simulink model "slip_regulation_stage2"  (R2018a)
settings: Solver=ode4  StartTime=0.0  StopTime=100  FixedStep=0.001  RelTol=1e-3
values from neighbouring files (symbols this model uses):
  B0 = 2.5    [init_params.m]
  Is = 0.2    [init_params.m]
  m = 100    [init_params.m]
  MFC1 = [9.5 1.9 1.14  0.75]    [init_params.m]
  MFC2 = [2.5 1.8 1 0.2]    [init_params.m]
  MFC3 = [1.5 1.8 0.4 0.2]    [init_params.m]
  N = 500    [init_params.m]
  r = 0.2    [init_params.m]
  v0 = 1    [init_params.m]
libraries: simulink x1
settings Model: Creator=obrusvit  LastModifiedBy=obrusvit

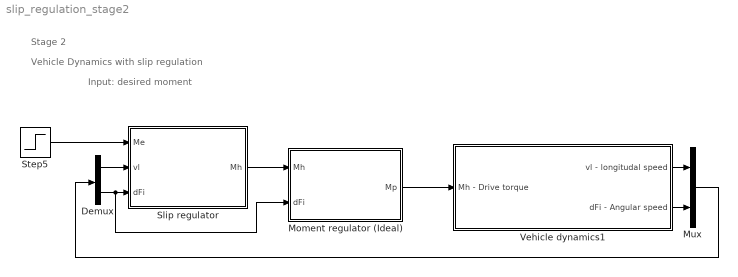
== system slip_regulation_stage2 ==
  note: Stage 2
  note: Input: desired moment
  note: Vehicle Dynamics with slip regulation
  Demux : Demux  Outputs=2
  Moment regulator (Ideal) : Subsystem
  Mux : Mux  Inputs=2
  Slip regulator : Subsystem
  Step5 : Step  Time=0  After=125  SampleTime=0
  Vehicle dynamics1 : Subsystem
  wires:
  Moment regulator (Ideal)/1("Mp ") -> Vehicle dynamics1/1(Mh - Drive torque)
  Slip regulator/1("Mh ") -> Moment regulator (Ideal)/1(Mh)
  Vehicle dynamics1/2(dFi - Angular speed) -> Mux/2
  Step5/1 -> Slip regulator/1(Me)
  Vehicle dynamics1/1(vl - longitudal speed) -> Mux/1
  Mux/1 -> Demux/1
  Demux/1 -> Slip regulator/2(vl)
  Demux/2 -> Moment regulator (Ideal)/2(dFi), Slip regulator/3(dFi)

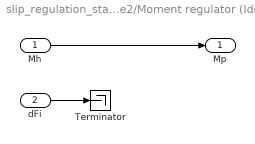
== system slip_regulation_stage2/Moment regulator (Ideal) ==
  Mh : Inport
  dFi : Inport  Port=2
  Terminator : Terminator
  "Mp " : Outport
  wires:
  Mh/1 -> "Mp "/1
  dFi/1 -> Terminator/1

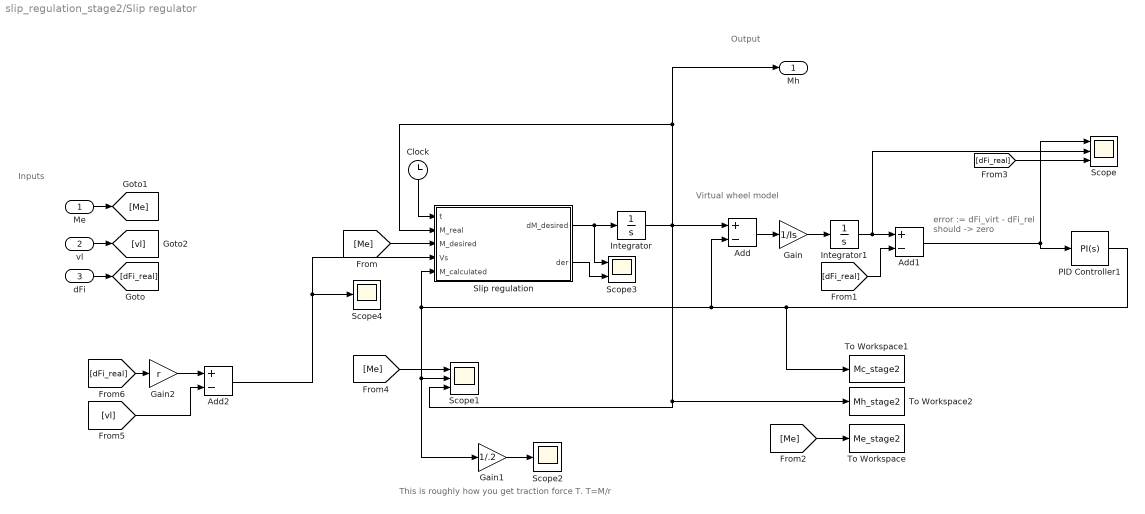
== system slip_regulation_stage2/Slip regulator ==
  note: This is roughly how you get traction force T. T=M/r
  note: error := dFi_virt - dFi_rel
      | should -> zero
  note: Virtual wheel model
  note: Output
  note: Inputs
  Me : Inport
  vl : Inport  Port=2
  dFi : Inport  Port=3
  Add : Sum  Inputs=+-
  Add1 : Sum  Inputs=+-
  Add2 : Sum  Inputs=+-
  Clock : Clock
  Gain : Gain  Gain=1/Is
  Gain1 : Gain  Gain=1/.2
  Gain2 : Gain  Gain=r
  Integrator : Integrator  LimitOutput=on  LowerSaturationLimit=0
  Integrator1 : Integrator
  PID Controller1 : simulink/Continuous/PID Controller  Controller=PI  TimeDomain=Continuous-time  SampleTime=-1  IntegratorMethod=Forward Euler  FilterMethod=Forward Euler  Form=Parallel  UseFilter=on  ControllerParametersSource=internal  P=15  I=20  D=0  N=100  InitialConditionSource=internal  InitialConditionForIntegrator=0  InitialConditionForFilter=0  ExternalReset=none  LimitOutput=on  UpperSaturationLimit=inf  LowerSaturationLimit=0  LinearizeAsGain=on  AntiWindupMode=none  Kb=1  TrackingMode=off  Kt=1  PParamMin=[]  PParamMax=[]  IParamMin=[]  IParamMax=[]  DParamMin=[]  DParamMax=[]  NParamMin=[]  NParamMax=[]  KbParamMin=[]  KbParamMax=[]  KtParamMin=[]  KtParamMax=[]  POutMin=[]  POutMax=[]  IOutMin=[]  IOutMax=[]  DOutMin=[]  DOutMax=[]  NOutMin=[]  NOutMax=[]  KbOutMin=[]  KbOutMax=[]  KtOutMin=[]  KtOutMax=[]  IntegratorOutMin=[]  IntegratorOutMax=[]  FilterOutMin=[]  FilterOutMax=[]  SumOutMin=[]  SumOutMax=[]  SumI1OutMin=[]  SumI1OutMax=[]  SumI2OutMin=[]  SumI2OutMax=[]  SumI3OutMin=[]  SumI3OutMax=[]  SumDOutMin=[]  SumDOutMax=[]  SaturationOutMin=[]  SaturationOutMax=[]  IntegratorContinuousStateAttributes=''  IntegratorStateMustResolveToSignalObject=off  IntegratorRTWStateStorageClass=Auto  FilterContinuousStateAttributes=''  FilterStateMustResolveToSignalObject=off  FilterRTWStateStorageClass=Auto  DifferentiatorICPrevScaledInput=0  DifferentiatorOutMin=[]  DifferentiatorOutMax=[]  FilterDiffOutCoefMin=[]  FilterDiffOutCoefMax=[]  SumDenOutMin=[]  SumDenOutMax=[]  SumNumOutMin=[]  SumNumOutMax=[]  ReciprocalOutMin=[]  ReciprocalOutMax=[]  DivideOutMin=[]  DivideOutMax=[]  TunerSelectOption=Transfer Function Based (PID Tuner App)
  Scope : Scope  NumInputPorts=3
  Scope1 : Scope  NumInputPorts=3
  Scope2 : Scope
  Scope3 : Scope  NumInputPorts=2
  Scope4 : Scope
  Slip regulation : MATLAB Function  TreatAsAtomicUnit=on
  To Workspace : ToWorkspace  VariableName=Me_stage2  SaveFormat=Timeseries  SampleTime=-1
  To Workspace1 : ToWorkspace  VariableName=Mc_stage2  SaveFormat=Timeseries  SampleTime=-1
  To Workspace2 : ToWorkspace  VariableName=Mh_stage2  SaveFormat=Timeseries  SampleTime=-1
  "Mh " : Outport
  wires:
  dFi/1 -> [dFi_real]
  Me/1 -> [Me]
  [Me] -> Slip regulation/3(M_desired)
  Slip regulation/1(dM_desired) -> Integrator/1, Scope3/1
  Add/1 -> Gain/1
  Gain/1 -> Integrator1/1
  [dFi_real] -> Add1/2
  Add1/1 -> PID Controller1/1, Scope/1
  Integrator1/1 -> Scope/2, Add1/1
  [dFi_real] -> Scope/3
  PID Controller1/1 -> To Workspace1/1, Scope1/2, Gain1/1, Slip regulation/5(M_calculated), Add/2
  [Me] -> Scope1/1
  Gain1/1 -> Scope2/1
  vl/1 -> [vl]
  Gain2/1 -> Add2/1
  [vl] -> Add2/2
  Add2/1 -> Scope4/1, Slip regulation/4(Vs)
  Clock/1 -> Slip regulation/1(t)
  Slip regulation/2(der) -> Scope3/2
  Integrator/1 -> Slip regulation/2(M_real), "Mh "/1, To Workspace2/1, Scope1/3, Add/1
  [dFi_real] -> Gain2/1
  [Me] -> To Workspace/1

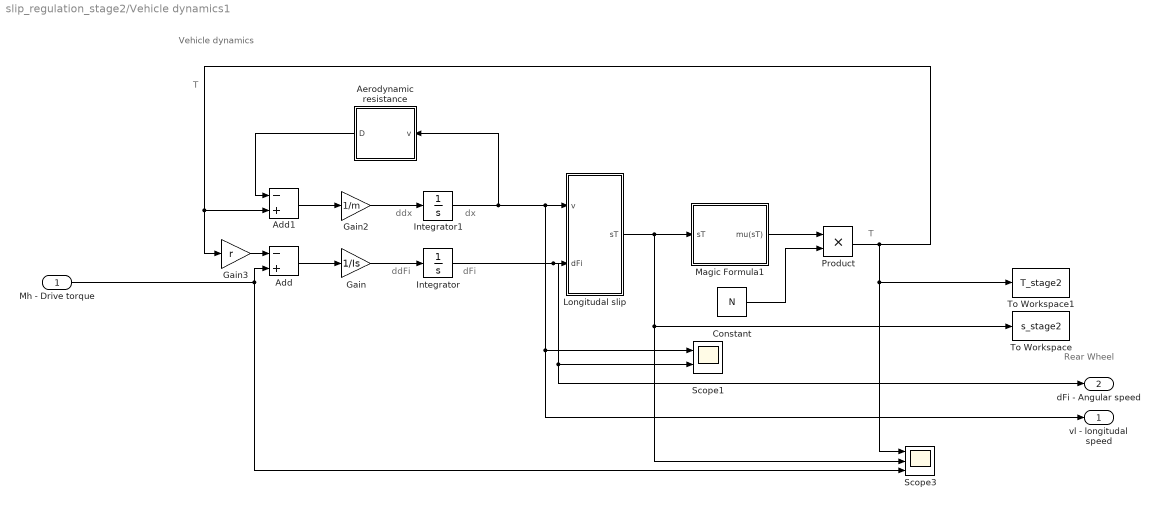
== system slip_regulation_stage2/Vehicle dynamics1 ==
  note: Vehicle dynamics
  note: Rear Wheel
  note: T
  note: ddx
  note: dx
  note: ddFi
  note: T
  note: dFi
  Mh - Drive torque : Inport
  Add : Sum  Inputs=-+
  Add1 : Sum  Inputs=-+
  "Aerodynamic resistance " : Subsystem
  Constant : Constant  Value=N
  Gain : Gain  Gain=1/Is
  Gain2 : Gain  Gain=1/m
  Gain3 : Gain  Gain=r
  Integrator : Integrator  InitialCondition=v0/r
  Integrator1 : Integrator  InitialCondition=v0
  Longitudal slip : Subsystem
  Magic Formula1 : Subsystem
  Product : Product
  Scope1 : Scope  NumInputPorts=2
  Scope3 : Scope  NumInputPorts=3
  To Workspace : ToWorkspace  VariableName=s_stage2  SaveFormat=Timeseries  SampleTime=-1
  To Workspace1 : ToWorkspace  VariableName=T_stage2  SaveFormat=Timeseries  SampleTime=-1
  vl - longitudal speed : Outport
  dFi - Angular speed : Outport  Port=2
  wires:
  Add1/1 -> Gain2/1
  Product/1 -> Gain3/1, Add1/2, To Workspace1/1, Scope3/1
  "Aerodynamic resistance "/1("D ") -> Add1/1
  Gain3/1 -> Add/1
  Magic Formula1/1(mu(sT)) -> Product/1
  Gain/1 -> Integrator/1
  Add/1 -> Gain/1
  Mh - Drive torque/1 -> Scope3/3, Add/2
  Constant/1 -> Product/2
  Gain2/1 -> Integrator1/1
  Integrator1/1 -> "Aerodynamic resistance "/1(v), Longitudal slip/1(v), vl - longitudal speed/1, Scope1/1
  Integrator/1 -> Scope1/2, dFi - Angular speed/1, Longitudal slip/2(dFi)
  Longitudal slip/1(sT) -> Scope3/2, To Workspace/1, Magic Formula1/1(sT)

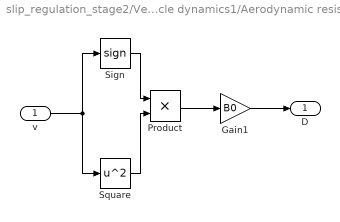
== system slip_regulation_stage2/Vehicle dynamics1/Aerodynamic resistance  ==
  v : Inport
  Gain1 : Gain  Gain=B0
  Product : Product
  Sign : Signum
  Square : Math  Operator=square  SaturateOnIntegerOverflow=on
  "D " : Outport
  wires:
  v/1 -> Sign/1, Square/1
  Square/1 -> Product/2
  Sign/1 -> Product/1
  Gain1/1 -> "D "/1
  Product/1 -> Gain1/1

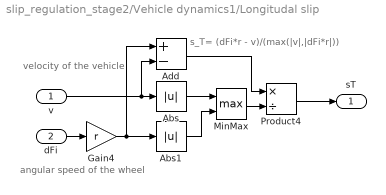
== system slip_regulation_stage2/Vehicle dynamics1/Longitudal slip ==
  note: s_T= (dFi*r - v)/(max(|v|,|dFi*r|))
  note: angular speed
      | of the wheel
  note: velocity
      | of the vehicle
  v : Inport
  dFi : Inport  Port=2
  Abs : Abs
  Abs1 : Abs
  Add : Sum  Inputs=+-
  Gain4 : Gain  Gain=r
  MinMax : MinMax  Function=max  Inputs=2
  Product4 : Product  Inputs=*/  RndMeth=Zero
  sT : Outport
  wires:
  Product4/1 -> sT/1
  Add/1 -> Product4/1
  Abs1/1 -> MinMax/2
  Abs/1 -> MinMax/1
  MinMax/1 -> Product4/2
  Gain4/1 -> Add/1, Abs1/1
  dFi/1 -> Gain4/1
  v/1 -> Add/2, Abs/1

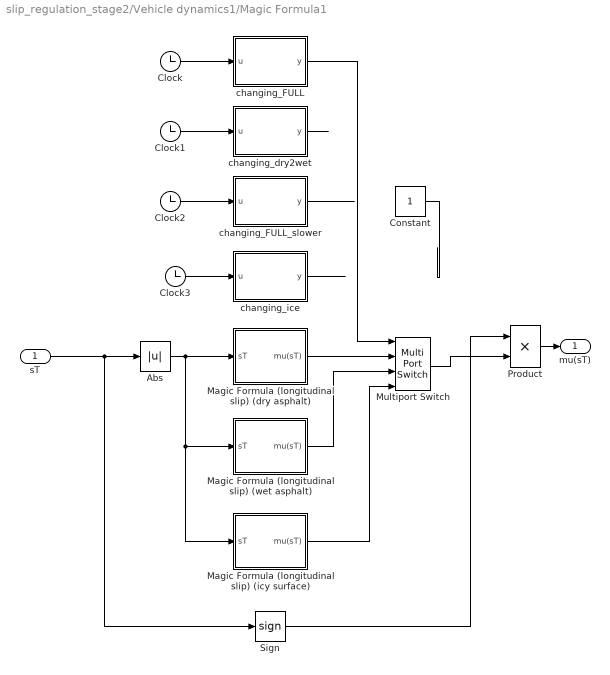
== system slip_regulation_stage2/Vehicle dynamics1/Magic Formula1 ==
  sT : Inport
  Abs : Abs
  Clock{,1..3} (4 alike) : Clock
  Constant : Constant
  Magic Formula (longitudinal slip) (dry asphalt) : Subsystem
  Magic Formula (longitudinal slip) (icy surface) : Subsystem
  Magic Formula (longitudinal slip) (wet asphalt) : Subsystem
  Multiport Switch : MultiPortSwitch
  Product : Product
  Sign : Signum
  changing_FULL : MATLAB Function  TreatAsAtomicUnit=on
  changing_FULL_slower : MATLAB Function  TreatAsAtomicUnit=on
  changing_dry2wet : MATLAB Function  TreatAsAtomicUnit=on
  changing_ice : MATLAB Function  TreatAsAtomicUnit=on
  mu(sT) : Outport
  wires:
  Abs/1 -> Magic Formula (longitudinal slip) (icy surface)/1(sT), Magic Formula (longitudinal slip) (wet asphalt)/1(sT), Magic Formula (longitudinal slip) (dry asphalt)/1(sT)
  Magic Formula (longitudinal slip) (dry asphalt)/1(mu(sT)) -> Multiport Switch/2
  Product/1 -> mu(sT)/1
  Sign/1 -> Product/1
  sT/1 -> Sign/1, Abs/1
  Magic Formula (longitudinal slip) (wet asphalt)/1(mu(sT)) -> Multiport Switch/3
  Multiport Switch/1 -> Product/2
  Magic Formula (longitudinal slip) (icy surface)/1(mu(sT)) -> Multiport Switch/4
  Clock/1 -> changing_FULL/1(u)
  changing_FULL/1(y) -> Multiport Switch/1
  Constant/1 -> ?
  Clock1/1 -> changing_dry2wet/1(u)
  changing_dry2wet/1(y) -> ?
  Clock2/1 -> changing_FULL_slower/1(u)
  changing_FULL_slower/1(y) -> ?
  changing_ice/1(y) -> ?
  Clock3/1 -> changing_ice/1(u)

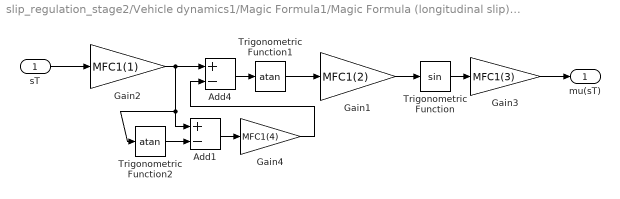
== system slip_regulation_stage2/Vehicle dynamics1/Magic Formula1/Magic Formula (longitudinal slip) (dry asphalt) ==
  sT : Inport
  Add1 : Sum  Inputs=+-
  Add4 : Sum  Inputs=+-
  Gain1 : Gain  Gain=MFC1(2)
  Gain2 : Gain  Gain=MFC1(1)
  Gain3 : Gain  Gain=MFC1(3)
  Gain4 : Gain  Gain=MFC1(4)
  Trigonometric Function : Trigonometry
  Trigonometric Function1 : Trigonometry  Operator=atan
  Trigonometric Function2 : Trigonometry  Operator=atan
  mu(sT) : Outport
  wires:
  Gain3/1 -> mu(sT)/1
  sT/1 -> Gain2/1
  Add4/1 -> Trigonometric Function1/1
  Gain4/1 -> Add4/2
  Add1/1 -> Gain4/1
  Trigonometric Function2/1 -> Add1/2
  Gain2/1 -> Trigonometric Function2/1, Add1/1, Add4/1
  Trigonometric Function1/1 -> Gain1/1
  Gain1/1 -> Trigonometric Function/1
  Trigonometric Function/1 -> Gain3/1

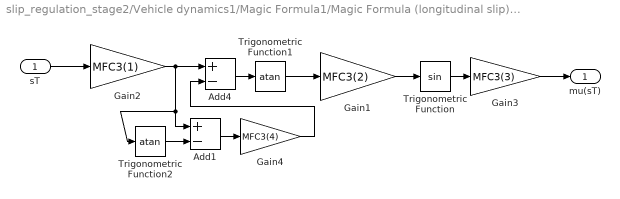
== system slip_regulation_stage2/Vehicle dynamics1/Magic Formula1/Magic Formula (longitudinal slip) (icy surface) ==
  sT : Inport
  Add1 : Sum  Inputs=+-
  Add4 : Sum  Inputs=+-
  Gain1 : Gain  Gain=MFC3(2)
  Gain2 : Gain  Gain=MFC3(1)
  Gain3 : Gain  Gain=MFC3(3)
  Gain4 : Gain  Gain=MFC3(4)
  Trigonometric Function : Trigonometry
  Trigonometric Function1 : Trigonometry  Operator=atan
  Trigonometric Function2 : Trigonometry  Operator=atan
  mu(sT) : Outport
  wires:
  Gain3/1 -> mu(sT)/1
  sT/1 -> Gain2/1
  Add4/1 -> Trigonometric Function1/1
  Gain4/1 -> Add4/2
  Add1/1 -> Gain4/1
  Trigonometric Function2/1 -> Add1/2
  Gain2/1 -> Trigonometric Function2/1, Add1/1, Add4/1
  Trigonometric Function1/1 -> Gain1/1
  Gain1/1 -> Trigonometric Function/1
  Trigonometric Function/1 -> Gain3/1

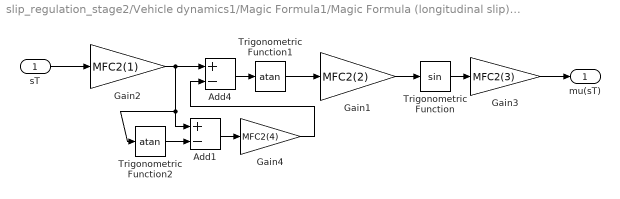
== system slip_regulation_stage2/Vehicle dynamics1/Magic Formula1/Magic Formula (longitudinal slip) (wet asphalt) ==
  sT : Inport
  Add1 : Sum  Inputs=+-
  Add4 : Sum  Inputs=+-
  Gain1 : Gain  Gain=MFC2(2)
  Gain2 : Gain  Gain=MFC2(1)
  Gain3 : Gain  Gain=MFC2(3)
  Gain4 : Gain  Gain=MFC2(4)
  Trigonometric Function : Trigonometry
  Trigonometric Function1 : Trigonometry  Operator=atan
  Trigonometric Function2 : Trigonometry  Operator=atan
  mu(sT) : Outport
  wires:
  Gain3/1 -> mu(sT)/1
  sT/1 -> Gain2/1
  Add4/1 -> Trigonometric Function1/1
  Gain4/1 -> Add4/2
  Add1/1 -> Gain4/1
  Trigonometric Function2/1 -> Add1/2
  Gain2/1 -> Trigonometric Function2/1, Add1/1, Add4/1
  Trigonometric Function1/1 -> Gain1/1
  Gain1/1 -> Trigonometric Function/1
  Trigonometric Function/1 -> Gain3/1

== matlab function slip_regulation_stage2/Vehicle dynamics1/Magic Formula1/changing_FULL ==
  data: u input; y output
function y = fcn(u)
if u <= 20
    y = 1;
elseif u <= 40
    y = 2;
elseif u <= 60
    y = 3;
elseif u <= 80
    y = 2;
else
    y = 1;
end
end

== matlab function slip_regulation_stage2/Slip regulator/Slip regulation ==
  settings: updateMethod=DISCRETE
  data: t input; M_real input; M_desired input; Vs input; dM_desired output; M_calculated input; der output
function [dM_desired, der] = fcn(t, M_real, M_desired, Vs, M_calculated)
dM_7 = 128;
dM_6 = 64;
dM_5 = 32;
dM_4 = 16;
dM_3 = 8;
dM_2 = 4;
dM_1 = 2;

ERR_TOLERABLE = 0.2;
Ts = 0.005;                  %sampling time of refreshing params and recomputing;
CRITICAL_SLIP_VEL = 10;
DERIV_THRESHOLD = 1;

persistent dT;
persistent dVs;

persistent last_Mcalc;
persistent last_Vs;

persistent last_t;

if isempty(dT)
    dT = M_calculated;
end
if isempty(dVs)
    dVs = 0;
end
if isempty(last_Mcalc)
    last_Mcalc = M_calculated;
end
if isempty(last_Vs)
    last_Vs = 0;
end
if isempty(last_t)
    last_t = t;
end
    

%% Main algorithm
if (t-last_t) >= Ts 
    
    % compute differences and save current values
    dT = M_calculated - last_Mcalc;
    dVs = Vs -last_Vs;
    last_t = t;
    last_Mcalc = M_calculated;
    last_Vs = Vs;

    diff = M_desired - M_calculated;
    der = 0;

    if abs(diff) <= ERR_TOLERABLE   %Force is just OK    
        dM_desired = 0;
    elseif diff <= ERR_TOLERABLE        %driver wants to REDUCE force
        dM_desired = -dM_4;
        %dM_desired = reduceForceForDriver(diff);
    else                                %driver wants to INCREASE force  
        if M_calculated == 0
            % get it runnin' booy
            dM_desired = dM_3;
            return
        end
        derivation = dT/dVs;
        der = derivation;
        dM_desired = choose_dM(derivation);
        if (Vs >= CRITICAL_SLIP_VEL)
            dM_desired = dM_desired - 1000;
        end
         if (M_calculated - M_real) >= 10
            % M_real is way below M_calc
            % that means we were slipping
            % but we do not want to drop M to zero
            dM_desired = 0;
        end
    end
else 
    dM_desired = 0;
    der = 0;
end

%     function dM_chosen = choose_dM(derivation)
%         if derivation >= DERIV_THRESHOLD
%             dM_chosen = dM_4;
%         else
%             dM_chosen = -dM_4;
%         end
%     end

    function dM_chosen = choose_dM(derivation)
        if derivation >= 50
            dM_chosen = dM_7;
        elseif derivation >= 20
            dM_chosen = dM_7;
        elseif derivation >= 8
            dM_chosen = dM_7;
        elseif derivation >= 4
            dM_chosen = dM_6; 
        elseif derivation >= 2
            dM_chosen = dM_5;
        elseif derivation >= DERIV_THRESHOLD
            dM_chosen = dM_4;
        elseif derivation >= 0.8
            dM_chosen = -dM_1;
        elseif derivation >= 0.6
            dM_chosen = -dM_2;
        elseif derivation >= 0.2
            dM_chosen = -dM_3;
        elseif derivation >= 0
            dM_chosen = -dM_4;
        elseif derivation >= -1
            dM_chosen = -dM_5;
        else
            %below zero
            dM_chosen = -dM_6;
        end
    end

end

== matlab function slip_regulation_stage2/Vehicle dynamics1/Magic Formula1/changing_dry2wet ==
  data: u input; y output
function y = fcn(u)
if u <= 100
    y = 1;
elseif u <= 200
    y = 2;
elseif u <= 300
    y = 1;
elseif u <= 400
    y = 2;
else
    y = 1;
end
end

== matlab function slip_regulation_stage2/Vehicle dynamics1/Magic Formula1/changing_FULL_slower ==
  data: u input; y output
function y = fcn(u)
if u <= 100
    y = 1;
elseif u<=200
    y = 2;
elseif u <= 300
    y = 3;
elseif u <= 400
    y = 2;
else
    y = 1;
end
end

== matlab function slip_regulation_stage2/Vehicle dynamics1/Magic Formula1/changing_ice ==
  data: u input; y output
function y = fcn(u)
if u <= 100
    y = 1;
elseif u <= 200
    y = 3;
else
    y = 3;
end
end
